simulink model "arm_sim"  (R2016b)
settings: Solver=ode45  StartTime=0.0  StopTime=10000  RelTol=1e-3  EnableMultiTasking=on
InitFcn:
  | addpath ./..
  | arm_param
libraries: simulink x1
settings Model: Creator=beard  LastModifiedBy=mclain
settings DataIOCC: LimitDataPoints=on  SaveFormat=Array  SignalLoggingSaveFormat=ModelDataLogs
settings OptimizationCC: ExpressionDepthLimit=2147483647  InitFltsAndDblsToZero=on  LifeSpan=inf
settings DebuggingCC: UnderspecifiedInitializationDetection=Classic  MergeDetectMultiDrivingBlocksExec=none  SolverPrmCheckMsg=warning  FcnCallInpInsideContextMsg=warning  StateNameClashWarn=warning  SFUnexpectedBacktrackingDiag=warning  SFNoUnconditionalDefaultTransitionDiag=warning  SFExecutionAtInitializationDiag=none
settings HardwareCC: ProdBitPerPointer=32  ProdBitPerSizeT=32  ProdBitPerPtrDiffT=32  ProdLargestAtomicFloat=None  ProdIntDivRoundTo=Undefined  ProdEndianess=Unspecified  ProdWordSize=32  ProdHWDeviceType=32-bit Generic
settings ModelReferenceCC: PropagateSignalLabelsOutOfModel=off
settings GRTTargetCC: TargetLangStandard=C89/C90 (ANSI)  GeneratePreprocessorConditionals=Disable all  CombineOutputUpdateFcns=off  GRTInterface=on
settings ConfigComp: CovMetricSettings=dw  CovHtmlReporting=on  CovSaveCumulativeToWorkspaceVar=on  CovSaveSingleToWorkspaceVar=on  CovExternalEMLEnable=off

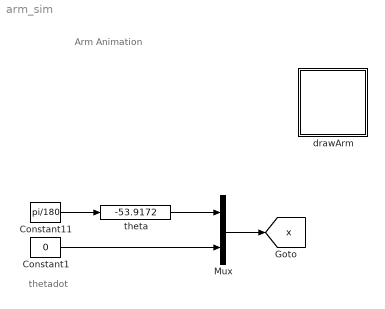
== system arm_sim ==
  note: thetadot
  note: Arm Animation
  Constant1 : Constant  Value=0
  Constant11 : Constant  Value=pi/180
  Mux : Mux  Inputs=2
  drawArm : Subsystem
      mask Display: image(imread('tv.jpg'))
  theta : simulink/Math Operations/Slider Gain  low=-180  gain=-53.9172  high=180
  tag scope: x=global
  wires:
  Constant11/1 -> theta/1
  theta/1 -> Mux/1
  Constant1/1 -> Mux/2
  Mux/1 -> [x]

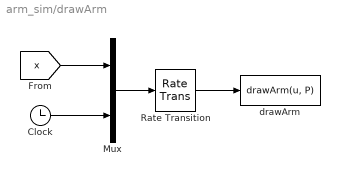
== system arm_sim/drawArm ==
  Clock : Clock
  Mux : Mux  Inputs=2
  Rate Transition : RateTransition  OutPortSampleTime=P.t_plot
  drawArm : MATLABFcn  MATLABFcn=drawArm(u, P)  OutputDimensions=0
  wires:
  [x] -> Mux/1
  Clock/1 -> Mux/2
  Mux/1 -> Rate Transition/1
  Rate Transition/1 -> drawArm/1
